simulink model "rate_contour"  (R2023a)
settings: Solver=VariableStepAuto  StartTime=0.0  StopTime=4  MaxStep=1e-4  RelTol=1e-3
values from neighbouring files (symbols this model uses):
  a_max = 1    [init_simulink.m]
  J = 3.29e-3    (= 0.00329)    [init_simulink.m]
  k_curr = 1    [init_simulink.m]
  k_pow = 10    [init_simulink.m]
  k_spd = 1    [init_simulink.m]
  ki_curr = (r_coeff * R) / (k_curr * k_pow)    (= 123.75)    [init_simulink.m]
  km = 0.98    [init_simulink.m]
  kp_curr = ki_curr * T_e    (= 0.8415)    [init_simulink.m]
  kw = 0.98    [init_simulink.m]
  R = 0.99    [init_simulink.m]
  t_accel = 0.8    [init_simulink.m]
  t_braking = 0.8    [init_simulink.m]
  t_const_rate = 1    [init_simulink.m]
  T_e = 0.0068    [init_simulink.m]
  T_pow = 0.0004    [init_simulink.m]
libraries: simulink x4
settings Model: Creator=k.balkunov  LastModifiedBy=k.balkunov

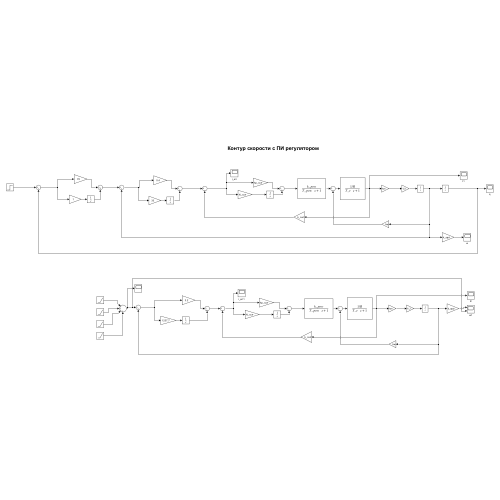
[thumbnail: Simulink's stored preview of the top-level diagram]
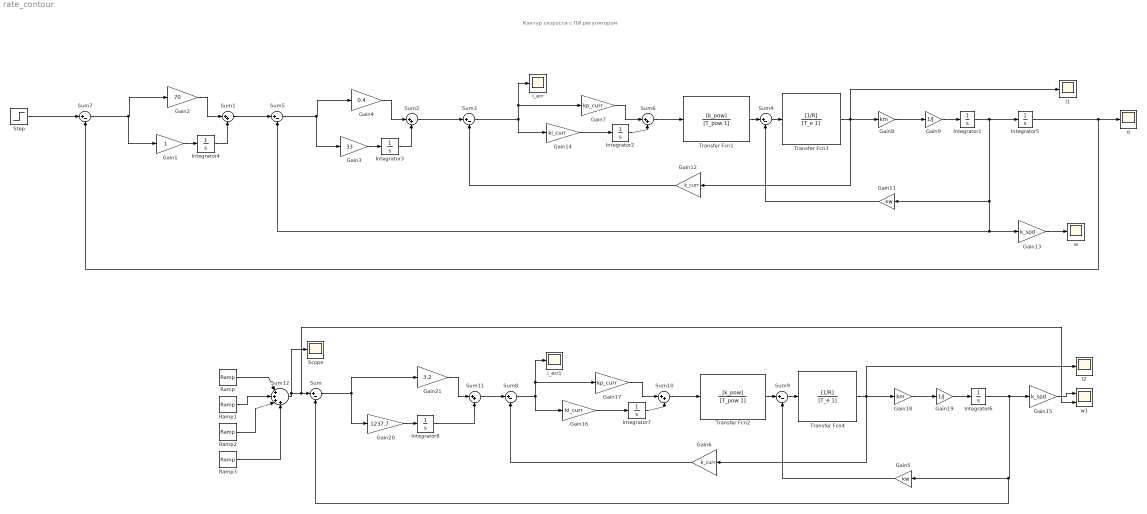
== system rate_contour ==
  note: Контур скорости с ПИ регулятором
  Gain1 : Gain
  Gain11 : Gain  Gain=kw
  Gain12 : Gain  Gain=k_curr
  Gain13 : Gain  Gain=k_spd
  Gain14 : Gain  Gain=ki_curr
  Gain15 : Gain  Gain=k_spd
  Gain16 : Gain  Gain=ki_curr
  Gain17 : Gain  Gain=kp_curr
  Gain18 : Gain  Gain=km
  Gain19 : Gain  Gain=1/J
  Gain2 : Gain  Gain=70
  Gain20 : Gain  Gain=1237.7
  Gain21 : Gain  Gain=3.2
  Gain3 : Gain  Gain=33
  Gain4 : Gain  Gain=0.4
  Gain5 : Gain  Gain=kw
  Gain6 : Gain  Gain=k_curr
  Gain7 : Gain  Gain=kp_curr
  Gain8 : Gain  Gain=km
  Gain9 : Gain  Gain=1/J
  I1 : Scope
  I2 : Scope
  Integrator{1..8} (8 alike) : Integrator
  Ramp : simulink/Sources/Ramp  slope=a_max  start=0  InitialOutput=0
  Ramp1 : simulink/Sources/Ramp  slope=-a_max  start=t_accel  InitialOutput=0
  Ramp2 : simulink/Sources/Ramp  slope=-a_max  start=t_accel + t_const_rate  InitialOutput=0
  Ramp3 : simulink/Sources/Ramp  slope=a_max  start=t_accel + t_const_rate + t_braking  InitialOutput=0
  Scope : Scope
  Step : Step  Time=0  SampleTime=0
  Sum{,3..5,7..9} (7 alike) : Sum  Inputs=|+-
  Sum{1..2,6,10..11} (5 alike) : Sum  Inputs=|++
  Sum12 : Sum  Inputs=|++++
  Transfer Fcn1 : TransferFcn  Numerator=[k_pow]  Denominator=[T_pow 1]
  Transfer Fcn2 : TransferFcn  Numerator=[k_pow]  Denominator=[T_pow 1]
  Transfer Fcn3 : TransferFcn  Numerator=[1/R]  Denominator=[T_e 1]
  Transfer Fcn4 : TransferFcn  Numerator=[1/R]  Denominator=[T_e 1]
  i_err : Scope
  i_err1 : Scope
  q : Scope
  w : Scope
  w1 : Scope  NumInputPorts=2
  wires:
  Sum2/1 -> Sum3/1
  Sum4/1 -> Transfer Fcn3/1
  Gain8/1 -> Gain9/1
  Gain13/1 -> w/1
  Gain11/1 -> Sum4/2
  Gain12/1 -> Sum3/2
  Transfer Fcn3/1 -> Gain8/1, Gain12/1, I1/1
  Integrator1/1 -> Integrator5/1, Sum5/2, Gain13/1, Gain11/1
  Sum6/1 -> Transfer Fcn1/1
  Sum3/1 -> i_err/1, Gain7/1, Gain14/1
  Gain7/1 -> Sum6/1
  Gain14/1 -> Integrator2/1
  Gain9/1 -> Integrator1/1
  Transfer Fcn1/1 -> Sum4/1
  Integrator2/1 -> Sum6/2
  Gain4/1 -> Sum2/1
  Integrator3/1 -> Sum2/2
  Gain3/1 -> Integrator3/1
  Sum5/1 -> Gain3/1, Gain4/1
  Gain2/1 -> Sum1/1
  Integrator4/1 -> Sum1/2
  Sum1/1 -> Sum5/1
  Gain1/1 -> Integrator4/1
  Sum7/1 -> Gain1/1, Gain2/1
  Integrator5/1 -> Sum7/2, q/1
  Step/1 -> Sum7/1
  Sum8/1 -> i_err1/1, Gain17/1, Gain16/1
  Transfer Fcn2/1 -> Sum9/1
  Integrator7/1 -> Sum10/2
  Gain16/1 -> Integrator7/1
  Gain17/1 -> Sum10/1
  Sum10/1 -> Transfer Fcn2/1
  Sum9/1 -> Transfer Fcn4/1
  Gain19/1 -> Integrator6/1
  Integrator6/1 -> Gain5/1, Sum/2, Gain15/1
  Gain18/1 -> Gain19/1
  Gain6/1 -> Sum8/2
  Sum11/1 -> Sum8/1
  Gain5/1 -> Sum9/2
  Gain15/1 -> w1/1
  Transfer Fcn4/1 -> Gain18/1, Gain6/1, I2/1
  Sum/1 -> Gain20/1, Gain21/1
  Gain21/1 -> Sum11/1
  Gain20/1 -> Integrator8/1
  Integrator8/1 -> Sum11/2
  Ramp/1 -> Sum12/1
  Ramp1/1 -> Sum12/2
  Ramp2/1 -> Sum12/3
  Ramp3/1 -> Sum12/4
  Sum12/1 -> Scope/1, w1/2, Sum/1
